simulink model "chuas_s"  (R2019a)
settings: Solver=FixedStepAuto  StartTime=0.0  StopTime=10  FixedStep=0.001  RelTol=1e-3
undefined symbols (not defined in the file or in its folder): a, b
settings Model: Creator=A  LastModifiedBy=86182
settings DataIOCC: SaveFormat=StructureWithTime
settings DebuggingCC: ArithmeticOperatorsInVariantConditions=warning
settings CodeAppCC: StateflowObjectComments=on

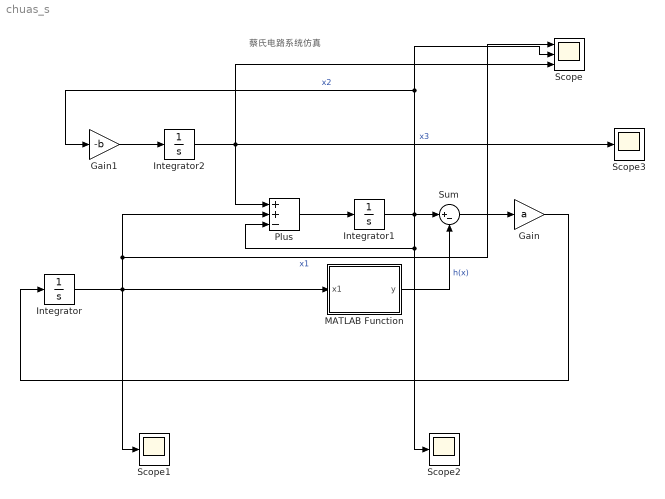
== system chuas_s ==
  note: 蔡氏电路系统仿真
  Gain : Gain  Gain=a
  Gain1 : Gain  Gain=-b
  Integrator : Integrator  InitialCondition=-0.1
  Integrator1 : Integrator  InitialCondition=0.1
  Integrator2 : Integrator  InitialCondition=0.2
  MATLAB Function : MATLAB Function  TreatAsAtomicUnit=on
  Plus : Sum  Inputs=++-
  Scope : Scope  NumInputPorts=3
  Scope1 : Scope
  Scope2 : Scope
  Scope3 : Scope
  Sum : Sum  Inputs=|+-
  wires:
  Integrator/1 -> Scope1/1, MATLAB Function/1(x1), Scope/1, Plus/2  "x1"
  MATLAB Function/1(y) -> Sum/2  "h(x)"
  Integrator1/1 -> Scope/2, Gain1/1, Sum/1, Scope2/1, Plus/3  "x2"
  Sum/1 -> Gain/1
  Gain/1 -> Integrator/1
  Integrator2/1 -> Scope/3, Plus/1, Scope3/1  "x3"
  Plus/1 -> Integrator1/1
  Gain1/1 -> Integrator2/1

== matlab function chuas_s/MATLAB Function ==
  data: x1 input; y output
function y = fcn(x1)
a=9;
b=14.28;
c=1;
m0=-(1/7);
m1=2/7;
c=1;

y = m1*x1+(1/2)*(m0-m1)*(abs(x1+c)-abs(x1-c));
